simulink model "example_of_logical_operator_and_bitwise_operator"  (R2021a)
settings: Solver=VariableStepAuto  StartTime=0.0  StopTime=10.0  RelTol=1e-3
libraries: simulink x4
settings Model: Creator=YasserNet  LastModifiedBy=YasserNet

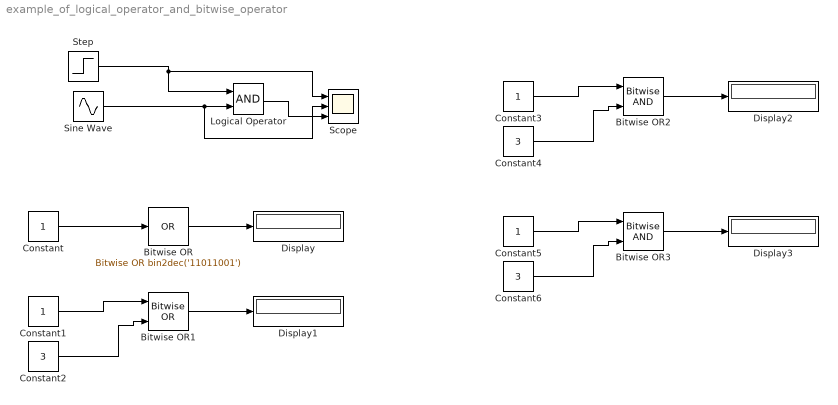
== system example_of_logical_operator_and_bitwise_operator ==
  Bitwise OR : simulink/Logic and Bit Operations/Bitwise Operator  logicop=OR  UseBitMask=on  BitMask=bin2dec('11011001')  BitMaskRealWorld=Stored Integer
  Bitwise OR1 : simulink/Logic and Bit Operations/Bitwise Operator  logicop=OR  UseBitMask=off  NumInputPorts=2  BitMask=bin2dec('11011001')  BitMaskRealWorld=Stored Integer
  Bitwise OR2 : simulink/Logic and Bit Operations/Bitwise Operator  logicop=AND  UseBitMask=off  NumInputPorts=2  BitMask=bin2dec('11011001')  BitMaskRealWorld=Stored Integer
  Bitwise OR3 : simulink/Logic and Bit Operations/Bitwise Operator  logicop=AND  UseBitMask=off  NumInputPorts=2  BitMask=bin2dec('11011001')  BitMaskRealWorld=Stored Integer
  Constant : Constant  OutDataTypeStr=int8
  Constant1 : Constant  OutDataTypeStr=int8
  Constant2 : Constant  Value=3  OutDataTypeStr=int8
  Constant3 : Constant  OutDataTypeStr=int8
  Constant4 : Constant  Value=3  OutDataTypeStr=int8
  Constant5 : Constant  OutDataTypeStr=int16
  Constant6 : Constant  Value=3  OutDataTypeStr=int16
  Display{,1..3} (4 alike) : Display
  Logical Operator : Logic  AllPortsSameDT=off  OutDataTypeStr=boolean
  Scope : Scope  NumInputPorts=3
  Sine Wave : Sin  Amplitude=5  Frequency=2*pi  SampleTime=0
  Step : Step  Time=3  SampleTime=0
  wires:
  Sine Wave/1 -> Scope/2, Logical Operator/2
  Logical Operator/1 -> Scope/3
  Step/1 -> Scope/1, Logical Operator/1
  Constant/1 -> Bitwise OR/1
  Bitwise OR/1 -> Display/1
  Bitwise OR1/1 -> Display1/1
  Constant1/1 -> Bitwise OR1/1
  Constant2/1 -> Bitwise OR1/2
  Constant4/1 -> Bitwise OR2/2
  Constant3/1 -> Bitwise OR2/1
  Bitwise OR2/1 -> Display2/1
  Bitwise OR3/1 -> Display3/1
  Constant5/1 -> Bitwise OR3/1
  Constant6/1 -> Bitwise OR3/2
